simulink model "ProjectFinal"  (R2019a)
settings: Solver=VariableStepAuto  StartTime=0.0  StopTime=10.0  RelTol=1e-3
values from neighbouring files (symbols this model uses):
  amplitude = str2num(get(handles.amp,'string'))    [finalGuiProject.m]    (also in open_short_test.m)
  frequency = str2num(get(handles.freq,'string'))    [finalGuiProject.m]    (also in open_short_test.m; stepDown.m; stepUp2.m)
  k = str2num(get(handles.a,'string'))    [finalGuiProject.m]
  L1 = str2num(get(handles.l1,'string'))    [finalGuiProject.m]
  L2 = str2num(get(handles.l2,'string'))    [finalGuiProject.m]
  Leq = sqrt((Vsc*Isc)^2-(Psc)^2)/((Isc^2)*2*pi*frequency)    [open_short_test.m]
  Ll = str2num(get(handles.ll,'string'))    [finalGuiProject.m]
  Lm = Voc^2/(sqrt((Voc*Ioc)^2-Poc^2)*2*pi*frequency)    [open_short_test.m]
  Lo = str2num(get(handles.lo,'string'))    [finalGuiProject.m]
  Nc = str2num(get(handles.nc,'string'))    [stepDown.m]    (also in stepUp2.m)
  Nse = str2num(get(handles.nse,'string'))    [stepDown.m]    (also in stepUp2.m)
  phase = str2num(get(handles.p,'string'))    [finalGuiProject.m]
  R1 = str2num(get(handles.r1,'string'))    [finalGuiProject.m]
  R2 = str2num(get(handles.r2,'string'))    [finalGuiProject.m]
  Req = Psc/Isc^2    [open_short_test.m]
  Rl = str2num(get(handles.rl,'string'))    [finalGuiProject.m]
  Rm = (Voc)^2/Poc    [open_short_test.m]
  Ro = str2num(get(handles.ro,'string'))    [finalGuiProject.m]
  S = str2num(get(handles.s,'string'))    [stepDown.m]    (also in stepUp2.m)
  Vh = str2num(get(handles.vh,'string'))    [stepDown.m]
  Vl = str2num(get(handles.vl,'string'))    [stepUp2.m]
libraries: fl_lib x15, nesl_utility x3
settings Model: Creator=HP  LastModifiedBy=HP

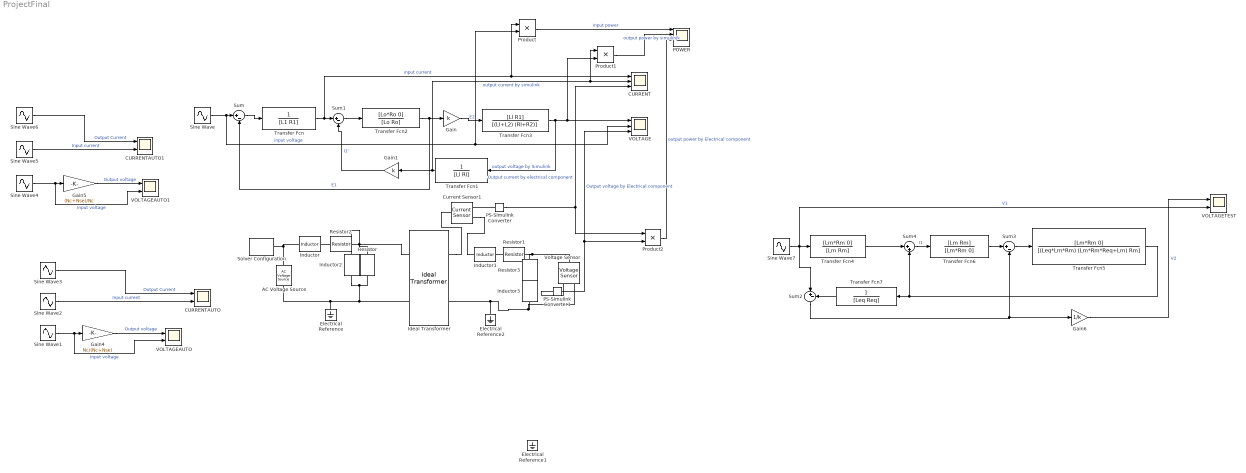
== system ProjectFinal ==
  AC Voltage Source : fl_lib/Electrical/Electrical Sources/AC Voltage Source  amp=amplitude V  shift=phase deg  frequency=frequency Hz  omega=0 rad/s
  CURRENT : Scope  NumInputPorts=3
  CURRENTAUTO : Scope  NumInputPorts=2
  CURRENTAUTO1 : Scope  NumInputPorts=2
  Current Sensor1 : fl_lib/Electrical/Electrical Sensors/Current Sensor
  Electrical Reference : fl_lib/Electrical/Electrical Elements/Electrical Reference
  Electrical Reference1 : fl_lib/Electrical/Electrical Elements/Electrical Reference
  Electrical Reference2 : fl_lib/Electrical/Electrical Elements/Electrical Reference
  Gain : Gain  Gain=k
  Gain1 : Gain  Gain=k
  Gain4 : Gain  Gain=Nc/(Nc+Nse)
  Gain5 : Gain  Gain=(Nc+Nse)/Nc
  Gain6 : Gain  Gain=1/k
  Ideal Transformer : fl_lib/Electrical/Electrical Elements/Ideal Transformer  n=1/k  i1_specify=off  i1_priority=None  i1=0 A  i1_nominal_specify=off  i1_nominal_unit=A  i1_nominal_value=1  v1_specify=off  v1_priority=None  v1=0 V  v1_nominal_specify=off  v1_nominal_unit=V  v1_nominal_value=1  i2_specify=off  i2_priority=None  i2=0 A  i2_nominal_specify=off  i2_nominal_unit=A  i2_nominal_value=1  v2_specify=off  v2_priority=None  v2=0 V  v2_nominal_specify=off  v2_nominal_unit=V  v2_nominal_value=1
      settings: SourceProductName=Simscape  SourceProductBaseCode=SS
  Inductor : fl_lib/Electrical/Electrical Elements/Inductor  l=L1 H  r=0 Ohm  g=0 1/Ohm  i_specify=off  i_priority=None  i=0 A  i_nominal_specify=off  i_nominal_unit=A  i_nominal_value=1  v_specify=off  v_priority=None  v=0 V  v_nominal_specify=off  v_nominal_unit=V  v_nominal_value=1  i_L_specify=off  i_L_priority=High  i_L=0 A  i_L_nominal_specify=off  i_L_nominal_unit=A  i_L_nominal_value=1
  Inductor1 : fl_lib/Electrical/Electrical Elements/Inductor  l=L2 H  r=0 Ohm  g=0 1/Ohm  i_specify=off  i_priority=None  i=0 A  i_nominal_specify=off  i_nominal_unit=A  i_nominal_value=1  v_specify=off  v_priority=None  v=0 V  v_nominal_specify=off  v_nominal_unit=V  v_nominal_value=1  i_L_specify=off  i_L_priority=High  i_L=0 A  i_L_nominal_specify=off  i_L_nominal_unit=A  i_L_nominal_value=1
  Inductor2 : fl_lib/Electrical/Electrical Elements/Inductor  l=Lo H  r=0 Ohm  g=0 1/Ohm  i_specify=off  i_priority=None  i=0 A  i_nominal_specify=off  i_nominal_unit=A  i_nominal_value=1  v_specify=off  v_priority=None  v=0 V  v_nominal_specify=off  v_nominal_unit=V  v_nominal_value=1  i_L_specify=off  i_L_priority=High  i_L=0 A  i_L_nominal_specify=off  i_L_nominal_unit=A  i_L_nominal_value=1
  Inductor3 : fl_lib/Electrical/Electrical Elements/Inductor  l=Ll H  r=0 Ohm  g=0 1/Ohm  i_specify=off  i_priority=None  i=0 A  i_nominal_specify=off  i_nominal_unit=A  i_nominal_value=1  v_specify=off  v_priority=None  v=0 V  v_nominal_specify=off  v_nominal_unit=V  v_nominal_value=1  i_L_specify=off  i_L_priority=High  i_L=0 A  i_L_nominal_specify=off  i_L_nominal_unit=A  i_L_nominal_value=1
  POWER : Scope  NumInputPorts=4
  PS-Simulink Converter : nesl_utility/PS-Simulink Converter  PhysicalDomain=network_engine_domain  SubClassName=ps_output  LeftPortType=input  RightPortType=output  PseudoPeriodic=off  Frequencies=[]  Unit=1  AffineConversion=off
  PS-Simulink Converter1 : nesl_utility/PS-Simulink Converter  PhysicalDomain=network_engine_domain  SubClassName=ps_output  LeftPortType=input  RightPortType=output  PseudoPeriodic=off  Frequencies=[]  Unit=1  AffineConversion=off
  Product : Product
  Product1 : Product
  Product2 : Product
  Resistor : fl_lib/Electrical/Electrical Elements/Resistor  R=Ro Ohm  i_specify=off  i_priority=None  i=0 A  i_nominal_specify=off  i_nominal_unit=A  i_nominal_value=1  v_specify=off  v_priority=None  v=0 V  v_nominal_specify=off  v_nominal_unit=V  v_nominal_value=1
  Resistor1 : fl_lib/Electrical/Electrical Elements/Resistor  R=R2 Ohm  i_specify=off  i_priority=None  i=0 A  i_nominal_specify=off  i_nominal_unit=A  i_nominal_value=1  v_specify=off  v_priority=None  v=0 V  v_nominal_specify=off  v_nominal_unit=V  v_nominal_value=1
  Resistor2 : fl_lib/Electrical/Electrical Elements/Resistor  R=R1 Ohm  i_specify=off  i_priority=None  i=0 A  i_nominal_specify=off  i_nominal_unit=A  i_nominal_value=1  v_specify=off  v_priority=None  v=0 V  v_nominal_specify=off  v_nominal_unit=V  v_nominal_value=1
  Resistor3 : fl_lib/Electrical/Electrical Elements/Resistor  R=Rl Ohm  i_specify=off  i_priority=None  i=0 A  i_nominal_specify=off  i_nominal_unit=A  i_nominal_value=1  v_specify=off  v_priority=None  v=0 V  v_nominal_specify=off  v_nominal_unit=V  v_nominal_value=1
  Sine Wave : Sin  Amplitude=amplitude  Frequency=frequency*2*pi  Phase=phase  SampleTime=0
  Sine Wave1 : Sin  Amplitude=Vh  Frequency=frequency*2*pi  SampleTime=0
  Sine Wave2 : Sin  Amplitude=S/Vh  Frequency=frequency*2*pi  SampleTime=0
  Sine Wave3 : Sin  Amplitude=S/(Vh*Nc/(Nc+Nse))  Frequency=frequency*2*pi  SampleTime=0
  Sine Wave4 : Sin  Amplitude=Vl  Frequency=frequency*2*pi  SampleTime=0
  Sine Wave5 : Sin  Amplitude=S/Vl  Frequency=frequency*2*pi  SampleTime=0
  Sine Wave6 : Sin  Amplitude=S/(Vl*(Nse+Nc)/Nc)  Frequency=frequency*2*pi  SampleTime=0
  Sine Wave7 : Sin  Amplitude=amplitude  Frequency=frequency*2*pi  SampleTime=0
  Solver Configuration : nesl_utility/Solver Configuration  PhysicalDomain=network_engine_domain  SubClassName=solver  LeftPortType=input  RightPortType=generic  Tones=[]  Harmonics=[]  SimulateNoise=off  Profile=off  UseLocalSampling=off  EnableSwitchedLinearOptims=on  FrequencyDomain=off  UseCCode=off  RelTol=0.001  AbsTol=1e-06  MinStep=1e-09  ToWorkspace=off  RevertToSquareIcSolve=off  NumHomotopyIterations=100  PhasorMode=off  PhasorModeNumHarmonics=1  DoDC=off  ResidualTolerance=1e-09  UseLocalSolver=off  LocalSolverChoice=NE_BACKWARD_EULER_ADVANCER  LocalSolverSampleTime=0.001  DoFixedCost=off  MaxNonlinIter=3  MaxModeIter=2  LinearAlgebra=auto  EquationFormulation=NE_TIME_EF  DelaysMemoryBudget=1024  AutomaticFiltering=on  FilteringTimeConstant=0.001  PartitionStorageMethod=AS_NEEDED  PartitionMemoryBudget=1024  PartitionMethod=ROBUST
  Sum{,1..3} (4 alike) : Sum  Inputs=|+-
  Sum4 : Sum  Inputs=|++
  Transfer Fcn : TransferFcn  Denominator=[L1 R1]
  Transfer Fcn1 : TransferFcn  Denominator=[Ll Rl]
  Transfer Fcn2 : TransferFcn  Numerator=[Lo*Ro 0]  Denominator=[Lo Ro]
  Transfer Fcn3 : TransferFcn  Numerator=[Ll R1]  Denominator=[(Ll+L2) (Rl+R2)]
  Transfer Fcn4 : TransferFcn  Numerator=[Lm*Rm 0]  Denominator=[Lm Rm]
  Transfer Fcn5 : TransferFcn  Numerator=[Lm*Rm 0]  Denominator=[(Leq*Lm*Rm) (Lm*Rm*Req+Lm) Rm]
  Transfer Fcn6 : TransferFcn  Numerator=[Lm Rm]  Denominator=[Lm*Rm 0]
  Transfer Fcn7 : TransferFcn  Denominator=[Leq Req]
  VOLTAGE : Scope  NumInputPorts=3
  VOLTAGEAUTO : Scope  NumInputPorts=2
  VOLTAGEAUTO1 : Scope  NumInputPorts=2
  VOLTAGETEST : Scope  NumInputPorts=2
  Voltage Sensor : fl_lib/Electrical/Electrical Sensors/Voltage Sensor
  wires:
  Sine Wave/1 -> VOLTAGE/2, Product/2, Sum/1  "input voltage"
  Sum/1 -> Transfer Fcn/1
  Transfer Fcn/1 -> Product/1, CURRENT/1, Sum1/1  "input current"
  Sum1/1 -> Transfer Fcn2/1
  Transfer Fcn2/1 -> Sum/2, Gain/1  "E1"
  Gain/1 -> Transfer Fcn3/1  "E2"
  Transfer Fcn3/1 -> Product1/2, VOLTAGE/1, Transfer Fcn1/1  "output voltage by Simulink"
  Transfer Fcn1/1 -> Product1/1, CURRENT/2, Gain1/1  "output current by simulink"
  Gain1/1 -> Sum1/2  "I1'"
  Product/1 -> POWER/1  "input power"
  Product1/1 -> POWER/2  "output power by simulinjk"
  PS-Simulink Converter1/1 -> Product2/2, VOLTAGE/3  "Output voltage by Electrical component"
  Product2/1 -> POWER/3  "output power by Electrical component"
  PS-Simulink Converter/1 -> Product2/1, CURRENT/3  "Output current by electrical component"
  Sine Wave1/1 -> VOLTAGEAUTO/2, Gain4/1  "Input voltage"
  Gain4/1 -> VOLTAGEAUTO/1  "Output voltage"
  Sine Wave2/1 -> CURRENTAUTO/2  "Input current"
  Sine Wave3/1 -> CURRENTAUTO/1  "Output Current"
  Sine Wave4/1 -> VOLTAGEAUTO1/2, Gain5/1  "Input voltage"
  Sine Wave5/1 -> CURRENTAUTO1/2  "Input current"
  Sine Wave6/1 -> CURRENTAUTO1/1  "Output Current"
  Gain5/1 -> VOLTAGEAUTO1/1  "Output voltage"
  Sine Wave7/1 -> Sum2/1, Transfer Fcn4/1, VOLTAGETEST/2  "V1"
  Transfer Fcn7/1 -> Sum2/2
  Transfer Fcn4/1 -> Sum4/1
  Sum4/1 -> Transfer Fcn6/1  "I1"
  Transfer Fcn6/1 -> Sum3/1
  Sum3/1 -> Transfer Fcn5/1
  Sum2/1 -> Gain6/1, Sum3/2
  Transfer Fcn5/1 -> Transfer Fcn7/1, Sum4/2
  Gain6/1 -> VOLTAGETEST/1  "V2"
  connections:
  AC Voltage Source/LConn1 -- Inductor/LConn1 -- Solver Configuration/RConn1
  Resistor2/LConn1 -- Inductor/RConn1
  Inductor2/LConn1 -- Resistor/LConn1 -- Ideal Transformer/LConn1 -- Resistor2/RConn1
  Electrical Reference/LConn1 -- AC Voltage Source/RConn1 -- Ideal Transformer/LConn2 -- Inductor2/RConn1 -- Resistor/RConn1
  Inductor3/LConn1 -- Resistor3/RConn1
  Inductor3/RConn1 -- Ideal Transformer/RConn2 -- Electrical Reference2/LConn1 -- Voltage Sensor/RConn2
  Inductor1/RConn1 -- Resistor1/LConn1
  Resistor1/RConn1 -- Resistor3/LConn1 -- Voltage Sensor/LConn1
  Voltage Sensor/RConn1 -- PS-Simulink Converter1/LConn1
  Ideal Transformer/RConn1 -- Current Sensor1/LConn1
  Current Sensor1/RConn2 -- Inductor1/LConn1
  PS-Simulink Converter/LConn1 -- Current Sensor1/RConn1
